simulink model "ballandbeamoff"  (R2018a)
settings: Solver=VariableStepAuto  StartTime=0.0  StopTime=10  RelTol=1e-3
values from neighbouring files (symbols this model uses):
  m = 0.15    [jacobianmat.m]
libraries: mblibv1 x12
settings Model: Creator=Hung Dung  LastModifiedBy=Hung Dung
settings SimMechanicsCC: VisOnUpdateDiagram=on  VisDuringSimulation=on

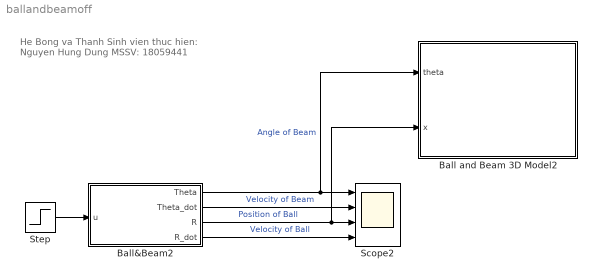
== system ballandbeamoff ==
  note: He Bong va Thanh
      | Sinh vien thuc hien: Nguyen Hung Dung
      | MSSV: 18059441
  Ball and Beam 3D Model2 : Subsystem
      mask Display: image(imread('3DModel.jpg'))
  Ball&Beam2 : Subsystem  mask{j1=1.5000e-05, j2=0.18, g=9.81, theta0=0, m=0.15, r0=0.05, R=0.03}
      mask prompts: j1 "moment quan tinh cua bong"; j2 "moment quan tinh cua thanh"; g "gia toc trong truong m/s^2"; theta0 "vi tri goc ban dau"; m "khoi luong bong"; r0 "vi tri bong ban dau"; R "ban kinh bong"
      mask DialogControl DescTextVar Prompt: He Bong va Thanh_SV: Nguyen Hung Dung 18059441
  Scope2 : Scope  NumInputPorts=4
  Step : Step  SampleTime=0
  wires:
  Step/1 -> Ball&Beam2/1(u)
  Ball&Beam2/1(Theta) -> Ball and Beam 3D Model2/1(theta), Scope2/1  "Angle of Beam"
  Ball&Beam2/3(R) -> Ball and Beam 3D Model2/2(x), Scope2/3  "Position of Ball"
  Ball&Beam2/4(R_dot) -> Scope2/4  "Velocity of Ball"
  Ball&Beam2/2(Theta_dot) -> Scope2/2  "Velocity of Beam"

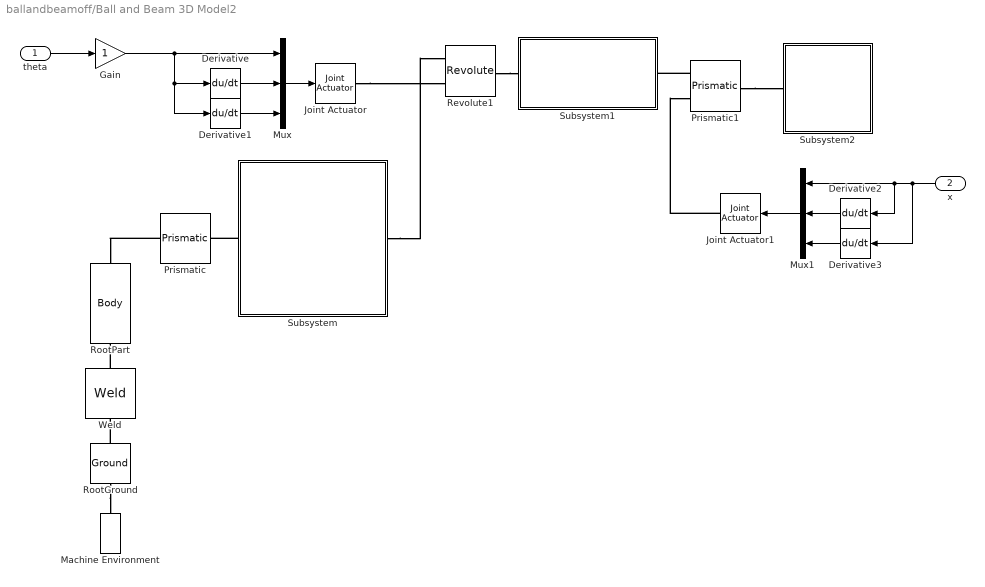
== system ballandbeamoff/Ball and Beam 3D Model2 ==
  theta : Inport
  x : Inport  Port=2
  Derivative{,1..3} (4 alike) : Derivative
  Gain : Gain
  Joint Actuator : mblibv1/Sensors &  Actuators/Joint Actuator  UpdateFromCAD=off  PhysicalDomain=Mechanical  PortType=blob  ActuationStyle=Motion  AngleUnits=rad  ArcVelocityUnits=rad/s  ArcAccelerationUnits=rad/s^2  CoordPositionUnits=m  VelocityUnits=m/s  AccelerationUnits=m/s^2  ForceUnits=N  TorqueUnits=N*m  ActiveIO=on  Width=3  DialogClass=MechanicalActuatorBlock  Primitive=R1  ReferenceFrame=Absolute (World)
      settings: SourceProductName=Simscape  SourceProductBaseCode=SS
  Joint Actuator1 : mblibv1/Sensors &  Actuators/Joint Actuator  UpdateFromCAD=off  PhysicalDomain=Mechanical  PortType=blob  ActuationStyle=Motion  AngleUnits=rad  ArcVelocityUnits=rad/s  ArcAccelerationUnits=rad/s^2  CoordPositionUnits=m  VelocityUnits=m/s  AccelerationUnits=m/s^2  ForceUnits=N  TorqueUnits=N*m  ActiveIO=on  Width=3  DialogClass=MechanicalActuatorBlock  Primitive=P1  ReferenceFrame=Absolute (World)
      settings: SourceProductName=Simscape  SourceProductBaseCode=SS
  Machine Environment : mblibv1/Bodies/Machine Environment  PortType=env  PhysicalDomain=Mechanical  DialogTemplateClass=MECH.MachineEnvironment  SyncWhenCopied=off  Gravity=[0 -9.81 0]  GravityUnits=m/s^2  GravityAsSignal=off  Dimensionality=Auto-detect  AnalysisType=Forward dynamics  LinearAssemblyTolerance=1e-3  LinearAssemblyToleranceUnits=m  AngularAssemblyTolerance=1e-3  AngularAssemblyToleranceUnits=rad  ConstraintSolverType=Stabilizing  ConstraintRelTolerance=1e-4  ConstraintAbsTolerance=1e-4  UseRobustSingularityHandling=off  RedundancyAnalysisToleranceType=Automatically select tolerance  RedundancyAnalysisTolerance=1e-14  StatePerturbationType=Fixed  PerturbationSize=1e-5  VisualizeMachine=on  BodyVisualizationType=Use model default body geometries  BodyColorSelMode=Use model default  DefaultBodyColor=[1 0 0]
      settings: SourceProductName=Simscape  SourceProductBaseCode=SS
  Mux : Mux  Inputs=3
  Mux1 : Mux  Inputs=3
  Prismatic : mblibv1/Joints/Prismatic  LConnTagsString=__newl0  RConnTagsString=__newr0  UpdateFromCAD=off  NumSAPorts=0  CutJoint=off  MarkAsCut=off  Primitives=prismatic  PrimitiveProps=P1$Base$[0 0 1]$prismatic  DialogClass=JointBlock  P1Axis=[0 0 1]
      settings: SourceProductName=Simscape  SourceProductBaseCode=SS
  Prismatic1 : mblibv1/Joints/Prismatic  LConnTagsString=__newl0|SA1  RConnTagsString=__newr0  UpdateFromCAD=off  NumSAPorts=1  CutJoint=off  MarkAsCut=off  Primitives=prismatic  PrimitiveProps=P1$Base$[1 0 0]$prismatic  DialogClass=JointBlock  P1Axis=[1 0 0]
      settings: SourceProductName=Simscape  SourceProductBaseCode=SS
  Revolute1 : mblibv1/Joints/Revolute  LConnTagsString=__newl0|SA1  RConnTagsString=__newr0  UpdateFromCAD=on  NumSAPorts=1  CutJoint=off  MarkAsCut=off  Primitives=prismatic  PrimitiveProps=R1$World$[0,0,1]$revolute  DialogClass=JointBlock  R1Axis=[0,0,1]
      settings: SourceProductName=Simscape  SourceProductBaseCode=SS
  RootGround : mblibv1/Bodies/Ground  UpdateFromCAD=on  LeftPortType=env  RightPortType=workingframe  PhysicalDomain=Mechanical  DialogClass=GroundBlock  CoordPosition=[7.39558e-007,-0.0451404,-0.0114254]  CoordPositionUnits=m  StateVectorMgrId=0  MachineId=[1 0]  ShowEnvPort=on  ParameterChecksum=[1627855958, 264127779, 2836122349, 3113692709]  TopologyChecksum=[2206919039, 2855131916, 2950705334, 2510259029]
      settings: SourceProductName=Simscape  SourceProductBaseCode=SS
  RootPart : mblibv1/Bodies/Body  LConnTagsString=CS4  RConnTagsString=CS2  UpdateFromCAD=on  DialogClass=MechanicalBodyBlock  Mass=0  MassUnits=kg  InertiaUnits=kg*m^2  Inertia=[0,0,0;0,0,0;0,0,0]  Shape=Cylinder  ShapeDims=[1 1]  ShapeUnits=m  ShapeUse=false  Density=1  DensityUnits=kg/m^3  DensityUse=false  GraphicsMode=MACHINE_DEFAULT  BodyColorSelMode=MACHINE_DEFAULT  BodyColor=[1 0 0]  AttachedToCS=CS1  CG=Right$CG$[7.39558e-007 -0.0451404 -0.0114254]$WORLD$WORLD$m$[1 0 0;0 1 0;0 0 1]$3x3 Transform$rad$WORLD$false$none  WorkingFrames=Right$CS1$[0 0 0]$WORLD$WORLD$m$[1 0 0;0 1 0;0 0 1]$3x3 Transform$rad$WORLD$false$none#Right$CS2$[0 0 0]$WORLD$WORLD$m$[1 0 0;0 1 0;0 0 1]$3x3 Transform$rad$WORLD$true$none#Left$CS3$[0 0 0]$WORLD$WORLD$m$[1 0 0;0 1 0;0 0 1]$3x3 Transform$rad$WORLD$false$none#Left$CS4$[7.39558e-007 -0.0451404 -0.0114254]$WORLD$WORLD$m$[1 0 0;0 1 0;0 0 1]$3x3 Transform$rad$WORLD$true$none#Right$CS5$[7.39558e-007 -0.0451404 -0.0114254]$WORLD$WORLD$m$[1 0 0;0 1 0;0 0 1]$3x3 Transform$rad$WORLD$false$none  CGPos=[7.39558e-007 -0.0451404 -0.0114254]  CGRot=[1 0 0;0 1 0;0 0 1]  CS0Pos=[]  CS0Rot=[]  CS1Pos=[0 0 0]  CS1Rot=[1 0 0;0 1 0;0 0 1]  CS2Pos=[0 0 0]  CS2Rot=[1 0 0;0 1 0;0 0 1]  CS3Pos=[0 0 0]  CS3Rot=[1 0 0;0 1 0;0 0 1]  CS4Pos=[7.39558e-007 -0.0451404 -0.0114254]  CS4Rot=[1 0 0;0 1 0;0 0 1]  CS5Pos=[7.39558e-007 -0.0451404 -0.0114254]  CS5Rot=[1 0 0;0 1 0;0 0 1]  CS6Pos=[]  CS6Rot=[]  CS7Pos=[]  CS7Rot=[]  CS8Pos=[]  CS8Rot=[]  CS9Pos=[]  CS9Rot=[]  CS10Pos=[]  CS10Rot=[]  CS11Pos=[]  CS11Rot=[]  CS12Pos=[]  CS12Rot=[]  CS13Pos=[]  CS13Rot=[]  CS14Pos=[]  CS14Rot=[]  CS15Pos=[]  CS15Rot=[]  CS16Pos=[]  CS16Rot=[]  CS17Pos=[]  CS17Rot=[]  CS18Pos=[]  CS18Rot=[]  CS19Pos=[]  CS19Rot=[]  CS20Pos=[]  CS20Rot=[]
      settings: SourceProductName=Simscape  SourceProductBaseCode=SS
  Subsystem : Subsystem
      mask Display: image(imread('BaseMotor.jpg'))
  Subsystem1 : Subsystem
      mask Display: image(imread('Beam.jpg'))
  Subsystem2 : Subsystem
      mask Display: image(imread('Ball.jpg'))
  Weld : mblibv1/Joints/Weld  LConnTagsString=__newl0  RConnTagsString=__newr0  UpdateFromCAD=on  NumSAPorts=0  CutJoint=off  MarkAsCut=off  Primitives=weld  PrimitiveProps=W$World$[0.57735,0.57735,0.57735]$weld  DialogClass=JointBlock  WAxis=[0.57735,0.57735,0.57735]
      settings: SourceProductName=Simscape  SourceProductBaseCode=SS
  wires:
  Mux/1 -> Joint Actuator/1
  theta/1 -> Gain/1
  Derivative/1 -> Mux/2
  Derivative1/1 -> Mux/3
  Mux1/1 -> Joint Actuator1/1
  Derivative2/1 -> Mux1/2
  Derivative3/1 -> Mux1/3
  x/1 -> Derivative3/1, Derivative2/1, Mux1/1
  Gain/1 -> Derivative1/1, Derivative/1, Mux/1
  connections:
  Joint Actuator1/RConn1 -- Prismatic1/LConn2
  Prismatic/LConn1 -- RootPart/RConn1
  Revolute1/RConn1 -- Subsystem1/LConn1
  RootGround/LConn1 -- Machine Environment/RConn1
  Subsystem/RConn1 -- Revolute1/LConn1
  Prismatic1/LConn1 -- Subsystem1/RConn1
  Joint Actuator/RConn1 -- Revolute1/LConn2
  RootGround/RConn1 -- Weld/LConn1
  Weld/RConn1 -- RootPart/LConn1
  Subsystem/LConn1 -- Prismatic/RConn1
  Prismatic1/RConn1 -- Subsystem2/LConn1

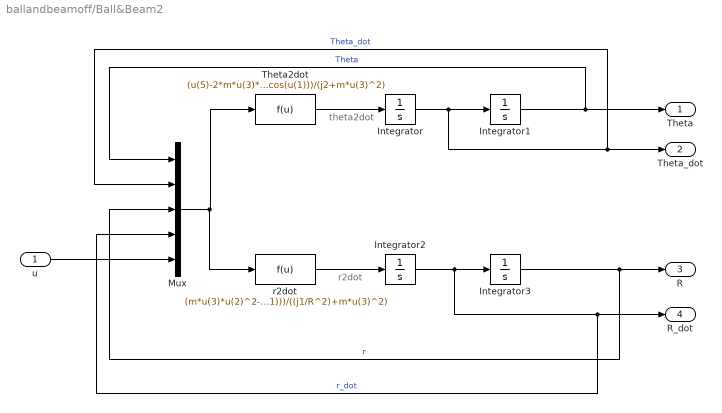
== system ballandbeamoff/Ball&Beam2 ==
  note: r2dot
  note: theta2dot
  u : Inport
  Integrator : Integrator
  Integrator1 : Integrator  InitialCondition=theta0
  Integrator2 : Integrator
  Integrator3 : Integrator  InitialCondition=r0
  Mux : Mux  Inputs=5
  "Theta2dot " : Fcn  Expr=(u(5)-2*m*u(3)*u(4)*u(2)-m*g*u(3)*cos(u(1)))/(j2+m*u(3)^2)
  "r2dot " : Fcn  Expr=(m*u(3)*u(2)^2-m*g*sin(u(1)))/((j1/R^2)+m*u(3)^2)
  Theta : Outport
  Theta_dot : Outport  Port=2
  R : Outport  Port=3
  R_dot : Outport  Port=4
  wires:
  "Theta2dot "/1 -> Integrator/1
  Integrator/1 -> Mux/2, Theta_dot/1, Integrator1/1  "Theta_dot"
  Mux/1 -> "r2dot "/1, "Theta2dot "/1
  "r2dot "/1 -> Integrator2/1
  Integrator2/1 -> R_dot/1, Mux/4, Integrator3/1  "r_dot"
  u/1 -> Mux/5
  Integrator1/1 -> Mux/1, Theta/1  "Theta"
  Integrator3/1 -> Mux/3, R/1  "r"

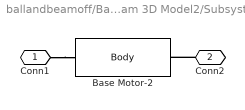
== system ballandbeamoff/Ball and Beam 3D Model2/Subsystem ==
  Base Motor-2 : mblibv1/Bodies/Body  LConnTagsString=CS3  RConnTagsString=CS2  UpdateFromCAD=on  DialogClass=MechanicalBodyBlock  Mass=0.336571  MassUnits=kg  InertiaUnits=kg*m^2  Inertia=[0.000801363,3.96141e-010,3.99171e-015;3.96141e-010,0.000314607,0.000206003;3.99171e-015,0.000206003,0.000797116]  Shape=Cylinder  ShapeDims=[1 1]  ShapeUnits=m  ShapeUse=false  Density=1  DensityUnits=kg/m^3  DensityUse=false  GraphicsMode=GFXFILE  GraphicsFileName=BallBeam - Base Motor-1.STL  BodyColorSelMode=COLORPALETTE  BodyColor=[0.14902;0.14902;0.14902]  AttachedToCS=CS1  CG=Right$CG$[0 -0.0689193 -0.0170081]$WORLD$WORLD$m$[1 0 0;0 1 0;0 0 1]$3x3 Transform$rad$WORLD$false$none  WorkingFrames=Right$CS1$[0 0 -0.0592]$WORLD$WORLD$m$[1 0 0;0 1 0;0 0 1]$3x3 Transform$rad$WORLD$false$none#Right$CS2$[0 0 -0.00849566]$WORLD$WORLD$m$[1 0 0;0 1 0;0 0 1]$3x3 Transform$rad$WORLD$true$none#Left$CS3$[0 0 -0.0592]$WORLD$WORLD$m$[1 0 0;0 1 0;0 0 1]$3x3 Transform$rad$WORLD$true$none  CGPos=[0 -0.0689193 -0.0170081]  CGRot=[1 0 0;0 1 0;0 0 1]  CS0Pos=[]  CS0Rot=[]  CS1Pos=[0 0 -0.0592]  CS1Rot=[1 0 0;0 1 0;0 0 1]  CS2Pos=[0 0 -0.00849566]  CS2Rot=[1 0 0;0 1 0;0 0 1]  CS3Pos=[0 0 -0.0592]  CS3Rot=[1 0 0;0 1 0;0 0 1]  CS4Pos=[]  CS4Rot=[]  CS5Pos=[]  CS5Rot=[]  CS6Pos=[]  CS6Rot=[]  CS7Pos=[]  CS7Rot=[]  CS8Pos=[]  CS8Rot=[]  CS9Pos=[]  CS9Rot=[]  CS10Pos=[]  CS10Rot=[]  CS11Pos=[]  CS11Rot=[]  CS12Pos=[]  CS12Rot=[]  CS13Pos=[]  CS13Rot=[]  CS14Pos=[]  CS14Rot=[]  CS15Pos=[]  CS15Rot=[]  CS16Pos=[]  CS16Rot=[]  CS17Pos=[]  CS17Rot=[]  CS18Pos=[]  CS18Rot=[]  CS19Pos=[]  CS19Rot=[]  CS20Pos=[]  CS20Rot=[]
      settings: SourceProductName=Simscape  SourceProductBaseCode=SS
  Conn1 : PMIOPort  Side=Left
  Conn2 : PMIOPort  Port=2  Side=Right
  connections:
  Conn1/RConn1 -- Base Motor-2/LConn1
  Conn2/RConn1 -- Base Motor-2/RConn1

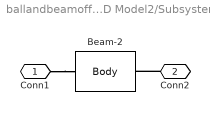
== system ballandbeamoff/Ball and Beam 3D Model2/Subsystem1 ==
  Beam-2 : mblibv1/Bodies/Body  LConnTagsString=CS2  RConnTagsString=CS3  UpdateFromCAD=on  DialogClass=MechanicalBodyBlock  Mass=0.142403  MassUnits=kg  InertiaUnits=kg*m^2  Inertia=[1.38091e-005,0,-8.90739e-011;0,0.00336681,1.14658e-009;-8.90739e-011,1.14658e-009,0.00337387]  Shape=Cylinder  ShapeDims=[1 1]  ShapeUnits=m  ShapeUse=false  Density=1  DensityUnits=kg/m^3  DensityUse=false  GraphicsMode=GFXFILE  GraphicsFileName=BallBeam - Beam-2.STL  BodyColorSelMode=COLORPALETTE  BodyColor=[0.2 0.4 1]  AttachedToCS=CS1  CG=Right$CG$[2.60119e-006 0.000607844 1.32563e-005]$WORLD$WORLD$m$[0.999991 0.00427933 0;-0.00427933 0.999991 0;0 0 1]$3x3 Transform$rad$WORLD$false$none  WorkingFrames=Left$CS1$[0 0 0]$WORLD$WORLD$m$[0.999991 0.00427933 0;-0.00427933 0.999991 0;0 0 1]$3x3 Transform$rad$WORLD$false$none#Left$CS2$[0 0 -0.00849566]$World$World$m$[1 0 0;0 1 0;0 0 1]$3x3 Transform$rad$WORLD$true$none#Right$CS3$[0 0.0228707 0]$CG$WORLD$m$[1 0 0;0 1 0;0 0 1]$3x3 Transform$rad$WORLD$true$none  CGPos=[2.60119e-006 0.000607844 1.32563e-005]  CGRot=[0.999991 0.00427933 0;-0.00427933 0.999991 0;0 0 1]  CS0Pos=[]  CS0Rot=[]  CS1Pos=[0 0 0]  CS1Rot=[0.999991 0.00427933 0;-0.00427933 0.999991 0;0 0 1]  CS2Pos=[0 0 -0.00849566]  CS2Rot=[1 0 0;0 1 0;0 0 1]  CS3Pos=[0 0.0228707 0]  CS3Rot=[1 0 0;0 1 0;0 0 1]  CS4Pos=[]  CS4Rot=[]  CS5Pos=[]  CS5Rot=[]  CS6Pos=[]  CS6Rot=[]  CS7Pos=[]  CS7Rot=[]  CS8Pos=[]  CS8Rot=[]  CS9Pos=[]  CS9Rot=[]  CS10Pos=[]  CS10Rot=[]  CS11Pos=[]  CS11Rot=[]  CS12Pos=[]  CS12Rot=[]  CS13Pos=[]  CS13Rot=[]  CS14Pos=[]  CS14Rot=[]  CS15Pos=[]  CS15Rot=[]  CS16Pos=[]  CS16Rot=[]  CS17Pos=[]  CS17Rot=[]  CS18Pos=[]  CS18Rot=[]  CS19Pos=[]  CS19Rot=[]  CS20Pos=[]  CS20Rot=[]
      settings: SourceProductName=Simscape  SourceProductBaseCode=SS
  Conn1 : PMIOPort  Side=Left
  Conn2 : PMIOPort  Port=2  Side=Right
  connections:
  Conn1/RConn1 -- Beam-2/LConn1
  Conn2/RConn1 -- Beam-2/RConn1

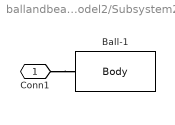
== system ballandbeamoff/Ball and Beam 3D Model2/Subsystem2 ==
  Ball-1 : mblibv1/Bodies/Body  LConnTagsString=CS1  UpdateFromCAD=on  DialogClass=MechanicalBodyBlock  Mass=0.0218881  MassUnits=kg  InertiaUnits=kg*m^2  Inertia=[6.70322e-007,0,0;0,6.70322e-007,0;0,0,6.70322e-007]  Shape=Cylinder  ShapeDims=[1 1]  ShapeUnits=m  ShapeUse=false  Density=1  DensityUnits=kg/m^3  DensityUse=false  GraphicsMode=GFXFILE  GraphicsFileName=BallBeam - Ball-1.STL  BodyColorSelMode=COLORPALETTE  BodyColor=[0.8 0.8 0.8]  AttachedToCS=CG  CG=Right$CG$[0 0.0228707 0]$Adjoining$World$m$[1 0 0;0 -1 0;0 0 -1]$3x3 Transform$rad$WORLD$false$none  WorkingFrames=Left$CS2$[0 0.0228707 0]$Adjoining$World$m$[1 0 0;0 1 0;0 0 1]$3x3 Transform$rad$WORLD$false$none#Left$CS1$[0 0 0]$Adjoining$Adjoining$m$[1 0 0;0 1 0;0 0 1]$3x3 Transform$rad$WORLD$true$none  CGPos=[0 0.0228707 0]  CGRot=[1 0 0;0 -1 0;0 0 -1]  CS0Pos=[]  CS0Rot=[]  CS1Pos=[0 0 0]  CS1Rot=[1 0 0;0 1 0;0 0 1]  CS2Pos=[0 0.0228707 0]  CS2Rot=[1 0 0;0 1 0;0 0 1]  CS3Pos=[]  CS3Rot=[]  CS4Pos=[]  CS4Rot=[]  CS5Pos=[]  CS5Rot=[]  CS6Pos=[]  CS6Rot=[]  CS7Pos=[]  CS7Rot=[]  CS8Pos=[]  CS8Rot=[]  CS9Pos=[]  CS9Rot=[]  CS10Pos=[]  CS10Rot=[]  CS11Pos=[]  CS11Rot=[]  CS12Pos=[]  CS12Rot=[]  CS13Pos=[]  CS13Rot=[]  CS14Pos=[]  CS14Rot=[]  CS15Pos=[]  CS15Rot=[]  CS16Pos=[]  CS16Rot=[]  CS17Pos=[]  CS17Rot=[]  CS18Pos=[]  CS18Rot=[]  CS19Pos=[]  CS19Rot=[]  CS20Pos=[]  CS20Rot=[]
      settings: SourceProductName=Simscape  SourceProductBaseCode=SS
  Conn1 : PMIOPort  Side=Left
  connections:
  Conn1/RConn1 -- Ball-1/LConn1
